simulink model "gm_sampleModel1420_3_sub"  (R2023a)
settings: Solver=VariableStepAuto  StartTime=0.0  StopTime=10.0  RelTol=1e-3
libraries: simulink x2, hdlsllib x2
settings Model: Creator=user1  LastModifiedBy=user1
settings OptimizationCC: BlockReduction=off  ConditionallyExecuteInputs=off
settings DebuggingCC: InheritedTsInSrcMsg=none

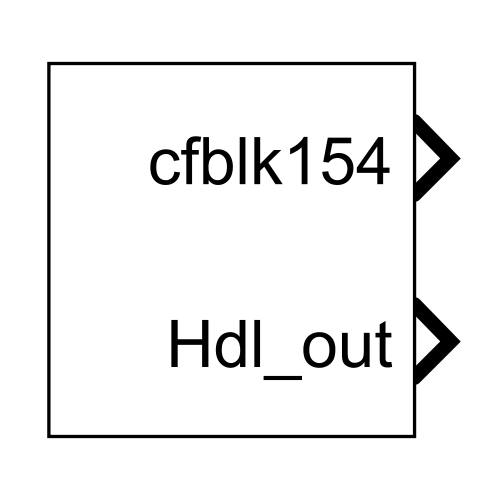
[thumbnail: Simulink's stored preview of the top-level diagram]
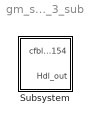
== system gm_sampleModel1420_3_sub ==
  Subsystem : Subsystem

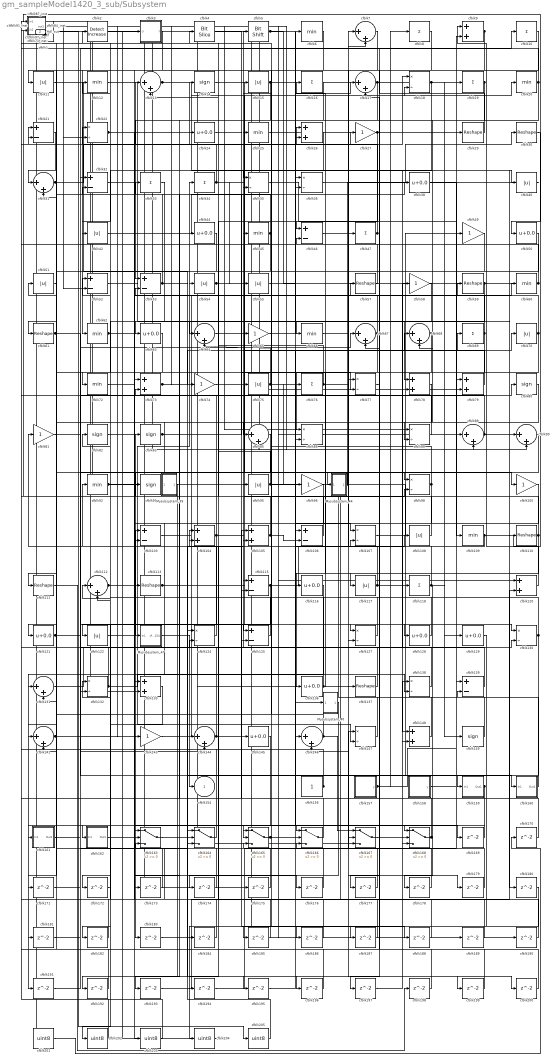
== system gm_sampleModel1420_3_sub/Subsystem ==
  Mysubsystem_39 : Subsystem
  Mysubsystem_40 : Subsystem
  Mysubsystem_44 : Subsystem
  Mysubsystem_47 : Subsystem
  cfblk1 : simulink/Logic and Bit Operations/Bit Clear  iBit=0
      settings: LibrarySourceBlock=|
      | hdlsllib/Logic and Bit
      | Operations/Bit Clear
  cfblk{8,10,16,19,33..34,47,69,76,118} (10 alike) : Sum  Inputs=+  OutDataTypeStr=uint8
  cfblk{27,49,58,65,74,81,96,100,143} (9 alike) : Gain  OutDataTypeStr=uint8
  cfblk102_inst : Subsystem
  cfblk{21,32,46,52..53,103,106,115,125,139} (10 alike) : Sum  Inputs=+-  OutDataTypeStr=uint8
  cfblk{9,26,73,78..79,104..105,120,133,148} (10 alike) : Sum  OutDataTypeStr=uint8
  cfblk{18,22,35..36,77,86,88,98,107,124,127,130,132,138,147} (15 alike) : Product  Inputs=*/  OutDataTypeStr=uint8  RndMeth=Zero  SaturateOnIntegerOverflow=on
  cfblk{11,15,40,42,51,54..55,70,75,95,108,117,122} (13 alike) : Abs  OutDataTypeStr=uint8  SaturateOnIntegerOverflow=off
  cfblk{6,12,20,25,45,60,62,66,72,92,109} (11 alike) : MinMax  OutDataTypeStr=uint8
  cfblk{29..30,57,59,61,110..111,113,137} (9 alike) : Reshape
  cfblk{7,13,17,31,64,67..68,85,89..90,112,131,141,144,146} (15 alike) : Sum  Inputs=|++  OutDataTypeStr=uint8
  cfblk114_inst : Subsystem
  cfblk{24,38,44,50,63,116,121,128..129,136,145} (11 alike) : Bias  Bias=0.0  SaturateOnIntegerOverflow=off
  cfblk119_inst : Subsystem
  cfblk135_inst : Subsystem
  cfblk{14,80,82..83,93,149} (6 alike) : Signum
  cfblk156 : Constant  OutDataTypeStr=uint8  SampleTime=-1
  cfblk157 : Subsystem  mask(Counter Limited){uplimit=double(7), tsamp=double(-1)}
      mask prompts: uplimit "Simulink:masks:UpperLimit_MP"; tsamp "Simulink:masks:SampleTime_MP"
      mask help: Simulink:masks:CounterLimited_MD
      mask init:
      | nbits = double(8);
      | tsamp = double(-1);
      | uplimit = double(7);
  cfblk158 : Subsystem  mask(Counter Free-Running){NumBits=double(16), tsamp=double(-1)}
      mask prompts: NumBits "Simulink:masks:NumberOfBits_MP"; tsamp "Simulink:masks:SampleTime_MP"
      mask help: Simulink:masks:CounterFreeRunning_MD
  cfblk159 : Subsystem
  cfblk160 : Subsystem
  cfblk161 : Subsystem
  cfblk162 : Subsystem
  cfblk{163..168} (6 alike) : Switch  OutDataTypeStr=uint8  SaturateOnIntegerOverflow=off  InputSameDT=off
  cfblk{169..200} (32 alike) : Delay  SampleTime=1
  cfblk2 : simulink/Logic and Bit Operations/Detect Increase  vinit=0.0  OutDataTypeStr=uint8
      settings: LibrarySourceBlock=|
      | hdlsllib/Logic and Bit
      | Operations/Detect
      | Increase
  cfblk{201..205} (5 alike) : DataTypeConversion  OutDataTypeStr=uint8  SaturateOnIntegerOverflow=off  RndMeth=Floor
  cfblk23_inst : Subsystem
  cfblk3 : Subsystem  mask(Detect Fall Negative){vinit=double(0), InputProcessing=Elements as channels (sample based), OutDataTypeStr=uint8}
      mask prompts: vinit "Simulink:masks:InitialCondition_MP"; InputProcessing "Simulink:masks:InputProcessing_MP"; OutDataTypeStr "Simulink:masks:OutputDataType_MP"
      mask help: Simulink:masks:DetectFallNegative_MD
      mask init:
      | InputProcessing = 'Elements as channels (sample based)';
      | OutDataTypeStr = 'uint8';
      | vinit = double(0);
      mask TypeOptions InputProcessing: Simulink:masks:ColumnsAsChannelsFrameBased | Simulink:masks:ElementsAsChannelsSampleBased
      mask TypeOptions OutDataTypeStr: Simulink:masks:uint8 | Simulink:masks:boolean
      mask Display: fprintf('U < 0\n&  NOT\nU/z < 0')
  cfblk4 : hdlsllib/Logic and Bit Operations/Bit Slice  lidx=7  ridx=0
  cfblk41_inst : Subsystem
  cfblk48_inst : Subsystem
  cfblk5 : hdlsllib/Logic and Bit Operations/Bit Shift  mode=Shift Left Logical  N=0
  cfblk56_inst : Subsystem
  cfblk71_inst : Subsystem
  cfblk84_inst : Subsystem
  cfblk87_inst : Subsystem
  cfblk91_inst : Subsystem
  cfblk97_inst : Subsystem
  cfblk154 : Outport  OutDataTypeStr=uint8  SampleTime=1  VectorParamsAs1DForOutWhenUnconnected=off
  Hdl_out : Outport  Port=2  OutDataTypeStr=uint8  SampleTime=1
  wires:
  Mysubsystem_39/1(Out1) -> cfblk192/1
  Mysubsystem_40/1(Out1) -> cfblk174/1
  Mysubsystem_44/1(Out1) -> cfblk183/1, cfblk159/1(In1)
  Mysubsystem_47/1(cfblk154) -> cfblk154/1
  cfblk1/1 -> cfblk205/1
  cfblk10/1 -> cfblk62/1
  cfblk100/1 -> cfblk143/1
  cfblk102_inst/1(out1) -> cfblk145/1, cfblk120/1
  cfblk103/1 -> cfblk57/1
  cfblk104/1 -> cfblk73/2, cfblk122/1, cfblk20/1
  cfblk105/1 -> cfblk5/1, cfblk106/2
  cfblk106/1 -> cfblk87_inst/2(in2)
  cfblk107/1 -> cfblk49/1
  cfblk108/1 -> cfblk52/1
  cfblk109/1 -> cfblk97_inst/1(in1), cfblk107/2
  cfblk11/1 -> cfblk164/2
  cfblk110/1 -> cfblk83/1, cfblk136/1
  cfblk111/1 -> cfblk198/1
  cfblk112/1 -> cfblk147/2, cfblk12/1, cfblk34/1
  cfblk113/1 -> cfblk128/1, cfblk98/2
  cfblk114_inst/1(out1) -> cfblk52/2
  cfblk115/1 -> cfblk7/2, cfblk162/1(In1)
  cfblk116/1 -> cfblk191/1
  cfblk117/1 -> cfblk58/1, cfblk2/1, cfblk92/1
  cfblk118/1 -> cfblk32/2, cfblk149/1, cfblk178/1
  cfblk119_inst/1(out1) -> cfblk201/1
  cfblk12/1 -> cfblk64/1
  cfblk120/1 -> cfblk9/1
  cfblk121/1 -> cfblk67/1, cfblk74/1
  cfblk122/1 -> cfblk103/1
  cfblk124/1 -> cfblk81/1
  cfblk125/1 -> cfblk71_inst/1(in1)
  cfblk127/1 -> cfblk87_inst/1(in1)
  cfblk128/1 -> cfblk106/1
  cfblk129/1 -> cfblk186/1
  cfblk13/1 -> cfblk180/1, cfblk18/2
  cfblk130/1 -> cfblk67/2, cfblk26/1, cfblk164/3
  cfblk131/1 -> cfblk78/2
  cfblk132/1 -> cfblk51/1, cfblk138/2
  cfblk133/1 -> cfblk172/1
  cfblk135_inst/1(out1) -> cfblk137/1
  cfblk136/1 -> cfblk95/1, cfblk200/1, cfblk16/1
  cfblk137/1 -> cfblk46/2
  cfblk138/1 -> cfblk82/1
  cfblk139/1 -> cfblk115/1
  cfblk14/1 -> cfblk148/1
  cfblk141/1 -> cfblk163/2, cfblk113/1
  cfblk143/1 -> cfblk47/1
  cfblk144/1 -> cfblk41_inst/2(in2), cfblk166/1
  cfblk145/1 -> cfblk202/1
  cfblk146/1 -> cfblk21/1, cfblk167/1, cfblk25/1
  cfblk147/1 -> cfblk102_inst/1(in1)
  cfblk148/1 -> cfblk104/1
  cfblk149/1 -> cfblk54/1
  cfblk15/1 -> cfblk40/1, cfblk193/1
  cfblk156/1 -> cfblk48_inst/2(in2), cfblk131/2
  cfblk157/1(y) -> cfblk9/2, cfblk8/1
  cfblk158/1(y) -> cfblk139/1
  cfblk159/1(Out1) -> cfblk182/1, cfblk181/1
  cfblk16/1 -> cfblk53/1
  cfblk160/1(Out1) -> cfblk139/2
  cfblk161/1(Out1) -> cfblk10/1
  cfblk162/1(Out1) -> cfblk27/1
  cfblk163/1 -> cfblk105/2
  cfblk164/1 -> cfblk84_inst/2(in2)
  cfblk165/1 -> cfblk70/1, cfblk108/1
  cfblk166/1 -> cfblk33/1
  cfblk167/1 -> cfblk138/1
  cfblk168/1 -> cfblk114_inst/2(in2), cfblk112/1
  cfblk169/1 -> cfblk165/2
  cfblk17/1 -> cfblk146/2, cfblk173/1
  cfblk170/1 -> cfblk105/1
  cfblk171/1 -> cfblk130/2
  cfblk172/1 -> cfblk132/1
  cfblk173/1 -> cfblk163/1
  cfblk174/1 -> cfblk112/2
  cfblk175/1 -> cfblk141/2
  cfblk176/1 -> cfblk124/2
  cfblk177/1 -> cfblk166/3
  cfblk178/1 -> cfblk147/1
  cfblk179/1 -> cfblk165/3
  cfblk18/1 -> cfblk42/1, cfblk129/1
  cfblk180/1 -> cfblk204/1
  cfblk181/1 -> cfblk144/2
  cfblk182/1 -> cfblk102_inst/2(in2)
  cfblk183/1 -> cfblk148/2
  cfblk184/1 -> cfblk163/3
  cfblk185/1 -> cfblk22/1
  cfblk186/1 -> cfblk84_inst/1(in1)
  cfblk187/1 -> cfblk26/2
  cfblk188/1 -> cfblk104/2
  cfblk189/1 -> cfblk73/1
  cfblk19/1 -> cfblk68/2, cfblk125/1
  cfblk190/1 -> cfblk21/2
  cfblk191/1 -> cfblk164/1
  cfblk192/1 -> cfblk23_inst/2(in2)
  cfblk193/1 -> cfblk120/2
  cfblk194/1 -> cfblk79/1
  cfblk195/1 -> cfblk146/1
  cfblk196/1 -> cfblk166/2
  cfblk197/1 -> cfblk168/3
  cfblk198/1 -> cfblk168/2
  cfblk199/1 -> cfblk17/2
  cfblk2/1 -> cfblk3/1(U)
  cfblk20/1 -> cfblk114_inst/1(in1), cfblk88/2
  cfblk200/1 -> cfblk31/2
  cfblk201/1 -> cfblk170/1
  cfblk202/1 -> cfblk119_inst/1(in1)
  cfblk203/1 -> cfblk119_inst/2(in2)
  cfblk204/1 -> cfblk1/1
  cfblk205/1 -> cfblk124/1
  cfblk21/1 -> cfblk31/1
  cfblk22/1 -> cfblk86/2, cfblk118/1
  cfblk23_inst/1(out1) -> cfblk167/3, cfblk144/1
  cfblk24/1 -> cfblk77/2
  cfblk25/1 -> Mysubsystem_40/1(In1)
  cfblk26/1 -> cfblk165/1
  cfblk27/1 -> cfblk46/1, cfblk184/1
  cfblk29/1 -> cfblk48_inst/1(in1)
  cfblk3/1(Y) -> cfblk203/1
  cfblk30/1 -> cfblk50/1
  cfblk31/1 -> cfblk7/1, cfblk14/1
  cfblk32/1 -> cfblk176/1
  cfblk33/1 -> cfblk63/1
  cfblk34/1 -> cfblk71_inst/2(in2), cfblk55/1, cfblk18/1
  cfblk35/1 -> cfblk89/1
  cfblk36/1 -> cfblk30/1
  cfblk38/1 -> cfblk109/1
  cfblk4/1 -> cfblk127/1
  cfblk40/1 -> Mysubsystem_39/1(In1)
  cfblk41_inst/1(out1) -> cfblk133/2
  cfblk42/1 -> cfblk6/1
  cfblk44/1 -> cfblk111/1
  cfblk45/1 -> cfblk97_inst/2(in2), cfblk103/2
  cfblk46/1 -> cfblk77/1
  cfblk47/1 -> cfblk91_inst/2(in2), cfblk13/1
  cfblk48_inst/1(out1) -> cfblk88/1, cfblk190/1
  cfblk49/1 -> cfblk187/1
  cfblk5/1 -> cfblk168/1, cfblk107/1
  cfblk50/1 -> cfblk85/1
  cfblk51/1 -> cfblk131/1
  cfblk52/1 -> cfblk110/1
  cfblk53/1 -> cfblk56_inst/1(in1), cfblk199/1
  cfblk54/1 -> cfblk38/1, cfblk188/1
  cfblk55/1 -> cfblk36/2
  cfblk56_inst/1(out1) -> cfblk90/1
  cfblk57/1 -> cfblk91_inst/1(in1)
  cfblk58/1 -> cfblk78/1
  cfblk59/1 -> cfblk197/1, cfblk72/1
  cfblk6/1 -> cfblk61/1
  cfblk60/1 -> cfblk41_inst/1(in1), Hdl_out/1
  cfblk61/1 -> cfblk160/1(In1), Mysubsystem_47/1(In1), Mysubsystem_44/1(In1)
  cfblk62/1 -> cfblk130/1, cfblk60/1
  cfblk63/1 -> cfblk161/1(In1)
  cfblk64/1 -> cfblk66/1
  cfblk65/1 -> cfblk17/1
  cfblk66/1 -> cfblk169/1
  cfblk67/1 -> cfblk15/1, cfblk115/2
  cfblk68/1 -> cfblk116/1, cfblk86/1
  cfblk69/1 -> cfblk4/1, cfblk35/2, cfblk194/1
  cfblk7/1 -> cfblk185/1
  cfblk70/1 -> cfblk53/2, cfblk141/1
  cfblk71_inst/1(out1) -> cfblk85/2, cfblk29/1, cfblk22/2
  cfblk72/1 -> cfblk196/1
  cfblk73/1 -> cfblk195/1, cfblk69/1
  cfblk74/1 -> cfblk68/1
  cfblk75/1 -> cfblk64/2, cfblk96/1
  cfblk76/1 -> cfblk13/2, cfblk179/1
  cfblk77/1 -> cfblk177/1
  cfblk78/1 -> cfblk171/1
  cfblk79/1 -> cfblk65/1
  cfblk8/1 -> cfblk117/1
  cfblk80/1 -> cfblk93/1
  cfblk81/1 -> cfblk80/1
  cfblk82/1 -> cfblk75/1
  cfblk83/1 -> cfblk59/1, cfblk36/1
  cfblk84_inst/1(out1) -> cfblk90/2, cfblk79/2
  cfblk85/1 -> cfblk121/1
  cfblk86/1 -> cfblk100/1
  cfblk87_inst/1(out1) -> cfblk89/2, cfblk175/1, cfblk19/1
  cfblk88/1 -> cfblk45/1
  cfblk89/1 -> cfblk56_inst/2(in2), cfblk32/1, cfblk135_inst/2(in2)
  cfblk9/1 -> cfblk11/1, cfblk35/1, cfblk127/2
  cfblk90/1 -> cfblk132/2
  cfblk91_inst/1(out1) -> cfblk189/1
  cfblk92/1 -> cfblk24/1, cfblk167/2
  cfblk93/1 -> cfblk23_inst/1(in1)
  cfblk95/1 -> cfblk44/1, cfblk98/1
  cfblk96/1 -> cfblk133/1
  cfblk97_inst/1(out1) -> cfblk76/1
  cfblk98/1 -> cfblk135_inst/1(in1), cfblk125/2

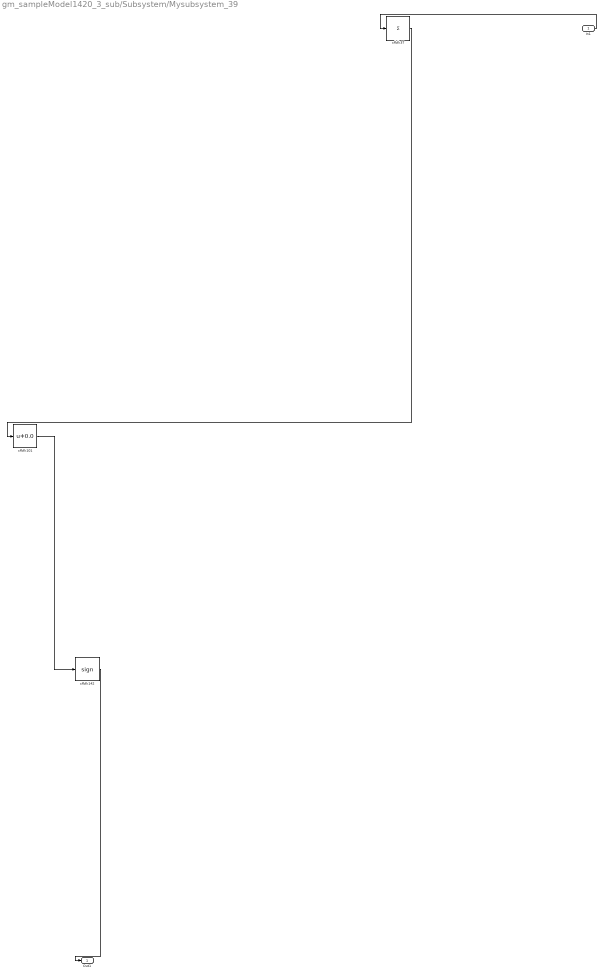
== system gm_sampleModel1420_3_sub/Subsystem/Mysubsystem_39 ==
  In1 : Inport  OutDataTypeStr=uint8  PortDimensions=1  SampleTime=1
  cfblk101 : Bias  Bias=0.0  SaturateOnIntegerOverflow=off
  cfblk142 : Signum
  cfblk37 : Sum  Inputs=+
  Out1 : Outport  SampleTime=1
  wires:
  In1/1 -> cfblk37/1
  cfblk101/1 -> cfblk142/1
  cfblk142/1 -> Out1/1
  cfblk37/1 -> cfblk101/1

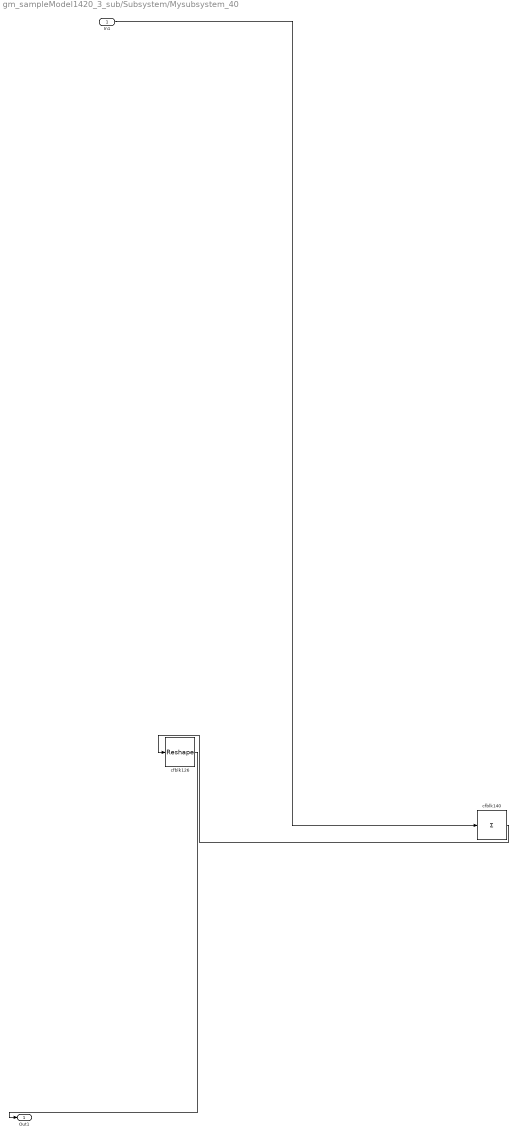
== system gm_sampleModel1420_3_sub/Subsystem/Mysubsystem_40 ==
  In1 : Inport  OutDataTypeStr=uint8  PortDimensions=1  SampleTime=1
  cfblk126 : Reshape
  cfblk140 : Sum  Inputs=+
  Out1 : Outport  SampleTime=1
  wires:
  In1/1 -> cfblk140/1
  cfblk126/1 -> Out1/1
  cfblk140/1 -> cfblk126/1

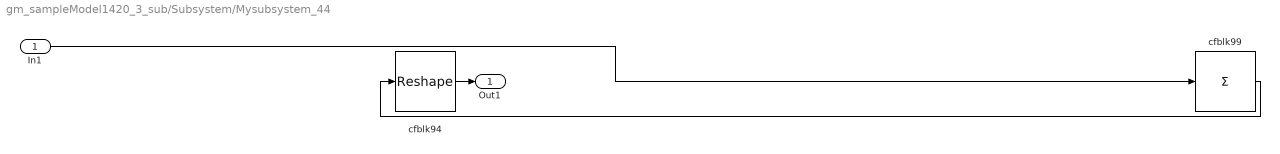
== system gm_sampleModel1420_3_sub/Subsystem/Mysubsystem_44 ==
  In1 : Inport  OutDataTypeStr=uint8  PortDimensions=1  SampleTime=1
  cfblk94 : Reshape
  cfblk99 : Sum  Inputs=+
  Out1 : Outport  SampleTime=1
  wires:
  In1/1 -> cfblk99/1
  cfblk94/1 -> Out1/1
  cfblk99/1 -> cfblk94/1

== system gm_sampleModel1420_3_sub/Subsystem/Mysubsystem_47 ==
  In1 : Inport  OutDataTypeStr=uint8  PortDimensions=1  SampleTime=1
  cfblk123 : Abs  SaturateOnIntegerOverflow=off
  cfblk154 : Outport  SampleTime=1  VectorParamsAs1DForOutWhenUnconnected=off
  wires:
  In1/1 -> cfblk123/1
  cfblk123/1 -> cfblk154/1

== system gm_sampleModel1420_3_sub/Subsystem/cfblk102_inst ==
  in1 : Inport  OutDataTypeStr=uint8  SampleTime=1
  in2 : Inport  Port=2  OutDataTypeStr=uint8  SampleTime=1
  mul_cfblk102_dotp_mulcomp : Product  Inputs=**  OutDataTypeStr=uint8  SampleTime=1
  out1 : Outport  OutDataTypeStr=uint8  SampleTime=1
  wires:
  in1/1 -> mul_cfblk102_dotp_mulcomp/1
  in2/1 -> mul_cfblk102_dotp_mulcomp/2
  mul_cfblk102_dotp_mulcomp/1 -> out1/1

== system gm_sampleModel1420_3_sub/Subsystem/cfblk114_inst ==
  in1 : Inport  OutDataTypeStr=uint8  SampleTime=1
  in2 : Inport  Port=2  OutDataTypeStr=uint8  SampleTime=1
  mul_cfblk114_dotp_mulcomp : Product  Inputs=**  OutDataTypeStr=uint8  SampleTime=1
  out1 : Outport  OutDataTypeStr=uint8  SampleTime=1
  wires:
  in1/1 -> mul_cfblk114_dotp_mulcomp/1
  in2/1 -> mul_cfblk114_dotp_mulcomp/2
  mul_cfblk114_dotp_mulcomp/1 -> out1/1

== system gm_sampleModel1420_3_sub/Subsystem/cfblk119_inst ==
  in1 : Inport  OutDataTypeStr=uint8  SampleTime=1
  in2 : Inport  Port=2  OutDataTypeStr=uint8  SampleTime=1
  mul_cfblk119_dotp_mulcomp : Product  Inputs=**  OutDataTypeStr=uint8  SampleTime=1
  out1 : Outport  OutDataTypeStr=uint8  SampleTime=1
  wires:
  in1/1 -> mul_cfblk119_dotp_mulcomp/1
  in2/1 -> mul_cfblk119_dotp_mulcomp/2
  mul_cfblk119_dotp_mulcomp/1 -> out1/1

== system gm_sampleModel1420_3_sub/Subsystem/cfblk135_inst ==
  in1 : Inport  OutDataTypeStr=uint8  SampleTime=1
  in2 : Inport  Port=2  OutDataTypeStr=uint8  SampleTime=1
  mul_cfblk135_dotp_mulcomp : Product  Inputs=**  OutDataTypeStr=uint8  SampleTime=1
  out1 : Outport  OutDataTypeStr=uint8  SampleTime=1
  wires:
  in1/1 -> mul_cfblk135_dotp_mulcomp/1
  in2/1 -> mul_cfblk135_dotp_mulcomp/2
  mul_cfblk135_dotp_mulcomp/1 -> out1/1

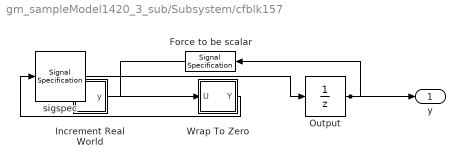
== system gm_sampleModel1420_3_sub/Subsystem/cfblk157 ==
  Force to be scalar : SignalSpecification  DisableCoverage=on  Dimensions=1
  Increment Real World : Subsystem  mask(Real World Value Increment){}
      mask help: Simulink:masks:RealWorldValueIncrement_MD
      mask Display: disp('V++')
  Output : UnitDelay  InitialCondition=0.0  SampleTime=tsamp  HasFrameUpgradeWarning=on
  Wrap To Zero : Subsystem  mask(Wrap To Zero){Threshold=double(7)}
      mask prompts: Threshold "Simulink:masks:Threshold_MP"
      mask help: Simulink:masks:WrapToZero_MD
  sigspec : SignalSpecification  OutDataTypeStr=uint8  Dimensions=1
  y : Outport  SampleTime=1
  wires:
  Force to be scalar/1 -> Increment Real World/1(u)
  Increment Real World/1(y) -> Wrap To Zero/1(U)
  Output/1 -> Force to be scalar/1, y/1
  Wrap To Zero/1(Y) -> sigspec/1
  sigspec/1 -> Output/1

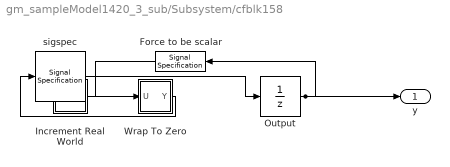
== system gm_sampleModel1420_3_sub/Subsystem/cfblk158 ==
  Force to be scalar : SignalSpecification  DisableCoverage=on  Dimensions=1
  Increment Real World : Subsystem  mask(Real World Value Increment){}
      mask help: Simulink:masks:RealWorldValueIncrement_MD
      mask Display: disp('V++')
  Output : UnitDelay  InitialCondition=0.0  SampleTime=tsamp  HasFrameUpgradeWarning=on
  Wrap To Zero : Subsystem  mask(Wrap To Zero){Threshold=double(65535)}
      mask prompts: Threshold "Simulink:masks:Threshold_MP"
      mask help: Simulink:masks:WrapToZero_MD
  sigspec : SignalSpecification  OutDataTypeStr=uint16  Dimensions=1
  y : Outport  SampleTime=1
  wires:
  Force to be scalar/1 -> Increment Real World/1(u)
  Increment Real World/1(y) -> Wrap To Zero/1(U)
  Output/1 -> Force to be scalar/1, y/1
  Wrap To Zero/1(Y) -> sigspec/1
  sigspec/1 -> Output/1

== system gm_sampleModel1420_3_sub/Subsystem/cfblk159 ==
  In1 : Inport  OutDataTypeStr=uint8  PortDimensions=1  SampleTime=1
  Out1 : Outport  SampleTime=1
  wires:
  In1/1 -> Out1/1

== system gm_sampleModel1420_3_sub/Subsystem/cfblk160 ==
  In1 : Inport  OutDataTypeStr=uint8  PortDimensions=1  SampleTime=1
  Out1 : Outport  SampleTime=1
  wires:
  In1/1 -> Out1/1

== system gm_sampleModel1420_3_sub/Subsystem/cfblk161 ==
  In1 : Inport  OutDataTypeStr=uint8  PortDimensions=1  SampleTime=1
  Out1 : Outport  SampleTime=1
  wires:
  In1/1 -> Out1/1

== system gm_sampleModel1420_3_sub/Subsystem/cfblk162 ==
  In1 : Inport  OutDataTypeStr=uint8  PortDimensions=1  SampleTime=1
  Out1 : Outport  SampleTime=1
  wires:
  In1/1 -> Out1/1

== system gm_sampleModel1420_3_sub/Subsystem/cfblk23_inst ==
  in1 : Inport  OutDataTypeStr=uint8  SampleTime=1
  in2 : Inport  Port=2  OutDataTypeStr=uint8  SampleTime=1
  mul_cfblk23_dotp_mulcomp : Product  Inputs=**  OutDataTypeStr=uint8  SampleTime=1
  out1 : Outport  OutDataTypeStr=uint8  SampleTime=1
  wires:
  in1/1 -> mul_cfblk23_dotp_mulcomp/1
  in2/1 -> mul_cfblk23_dotp_mulcomp/2
  mul_cfblk23_dotp_mulcomp/1 -> out1/1

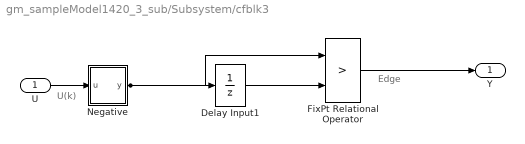
== system gm_sampleModel1420_3_sub/Subsystem/cfblk3 ==
  note: U(k)
  note: Edge
  U : Inport  OutDataTypeStr=uint8  SampleTime=1
  Delay Input1 : UnitDelay  Description=Store in Global RAM  DisableCoverage=on  InitialCondition=vinit  SampleTime=-1  HasFrameUpgradeWarning=on
  FixPt Relational Operator : RelationalOperator  Operator=>  OutDataTypeStr=fixdt(0, 8)  ZeroCross=off  InputSameDT=off
  Negative : Subsystem  mask(Compare To Zero){relop=<, OutDataTypeStr=boolean, ZeroCross=off}
      mask prompts: relop "Simulink:masks:Operator_MP"; OutDataTypeStr "Simulink:masks:OutputDataType_MP"; ZeroCross "Simulink:masks:EnableZerocrossingDetection_MP"
      mask help: Simulink:masks:CompareToZero_MD
      mask init:
      | OutDataTypeStr = 'boolean';
      | ZeroCross = 'off';
      | blkName = 'sampleModel1420_3_sub/Subsystem/cfblk3/Negative';
      | relop = '<';
      | setValue = 'boolean';
      mask TypeOptions relop: == | ~= | < | <= | >= | >
      mask TypeOptions OutDataTypeStr: Simulink:masks:uint8 | Simulink:masks:boolean
      mask Callback ZeroCross: sl('zeroCrossEnable', gcbh);
      mask Display: disp([relop,' 0'])
  Y : Outport  SampleTime=1
  wires:
  U/1 -> Negative/1(u)
  Delay Input1/1 -> FixPt Relational Operator/2
  FixPt Relational Operator/1 -> Y/1
  Negative/1(y) -> FixPt Relational Operator/1, Delay Input1/1

== system gm_sampleModel1420_3_sub/Subsystem/cfblk41_inst ==
  in1 : Inport  OutDataTypeStr=uint8  SampleTime=1
  in2 : Inport  Port=2  OutDataTypeStr=uint8  SampleTime=1
  mul_cfblk41_dotp_mulcomp : Product  Inputs=**  OutDataTypeStr=uint8  SampleTime=1
  out1 : Outport  OutDataTypeStr=uint8  SampleTime=1
  wires:
  in1/1 -> mul_cfblk41_dotp_mulcomp/1
  in2/1 -> mul_cfblk41_dotp_mulcomp/2
  mul_cfblk41_dotp_mulcomp/1 -> out1/1

== system gm_sampleModel1420_3_sub/Subsystem/cfblk48_inst ==
  in1 : Inport  OutDataTypeStr=uint8  SampleTime=1
  in2 : Inport  Port=2  OutDataTypeStr=uint8  SampleTime=1
  mul_cfblk48_dotp_mulcomp : Product  Inputs=**  OutDataTypeStr=uint8  SampleTime=1
  out1 : Outport  OutDataTypeStr=uint8  SampleTime=1
  wires:
  in1/1 -> mul_cfblk48_dotp_mulcomp/1
  in2/1 -> mul_cfblk48_dotp_mulcomp/2
  mul_cfblk48_dotp_mulcomp/1 -> out1/1

== system gm_sampleModel1420_3_sub/Subsystem/cfblk56_inst ==
  in1 : Inport  OutDataTypeStr=uint8  SampleTime=1
  in2 : Inport  Port=2  OutDataTypeStr=uint8  SampleTime=1
  mul_cfblk56_dotp_mulcomp : Product  Inputs=**  OutDataTypeStr=uint8  SampleTime=1
  out1 : Outport  OutDataTypeStr=uint8  SampleTime=1
  wires:
  in1/1 -> mul_cfblk56_dotp_mulcomp/1
  in2/1 -> mul_cfblk56_dotp_mulcomp/2
  mul_cfblk56_dotp_mulcomp/1 -> out1/1

== system gm_sampleModel1420_3_sub/Subsystem/cfblk71_inst ==
  in1 : Inport  OutDataTypeStr=uint8  SampleTime=1
  in2 : Inport  Port=2  OutDataTypeStr=uint8  SampleTime=1
  mul_cfblk71_dotp_mulcomp : Product  Inputs=**  OutDataTypeStr=uint8  SampleTime=1
  out1 : Outport  OutDataTypeStr=uint8  SampleTime=1
  wires:
  in1/1 -> mul_cfblk71_dotp_mulcomp/1
  in2/1 -> mul_cfblk71_dotp_mulcomp/2
  mul_cfblk71_dotp_mulcomp/1 -> out1/1

== system gm_sampleModel1420_3_sub/Subsystem/cfblk84_inst ==
  in1 : Inport  OutDataTypeStr=uint8  SampleTime=1
  in2 : Inport  Port=2  OutDataTypeStr=uint8  SampleTime=1
  mul_cfblk84_dotp_mulcomp : Product  Inputs=**  OutDataTypeStr=uint8  SampleTime=1
  out1 : Outport  OutDataTypeStr=uint8  SampleTime=1
  wires:
  in1/1 -> mul_cfblk84_dotp_mulcomp/1
  in2/1 -> mul_cfblk84_dotp_mulcomp/2
  mul_cfblk84_dotp_mulcomp/1 -> out1/1

== system gm_sampleModel1420_3_sub/Subsystem/cfblk87_inst ==
  in1 : Inport  OutDataTypeStr=uint8  SampleTime=1
  in2 : Inport  Port=2  OutDataTypeStr=uint8  SampleTime=1
  mul_cfblk87_dotp_mulcomp : Product  Inputs=**  OutDataTypeStr=uint8  SampleTime=1
  out1 : Outport  OutDataTypeStr=uint8  SampleTime=1
  wires:
  in1/1 -> mul_cfblk87_dotp_mulcomp/1
  in2/1 -> mul_cfblk87_dotp_mulcomp/2
  mul_cfblk87_dotp_mulcomp/1 -> out1/1

== system gm_sampleModel1420_3_sub/Subsystem/cfblk91_inst ==
  in1 : Inport  OutDataTypeStr=uint8  SampleTime=1
  in2 : Inport  Port=2  OutDataTypeStr=uint8  SampleTime=1
  mul_cfblk91_dotp_mulcomp : Product  Inputs=**  OutDataTypeStr=uint8  SampleTime=1
  out1 : Outport  OutDataTypeStr=uint8  SampleTime=1
  wires:
  in1/1 -> mul_cfblk91_dotp_mulcomp/1
  in2/1 -> mul_cfblk91_dotp_mulcomp/2
  mul_cfblk91_dotp_mulcomp/1 -> out1/1

== system gm_sampleModel1420_3_sub/Subsystem/cfblk97_inst ==
  in1 : Inport  OutDataTypeStr=uint8  SampleTime=1
  in2 : Inport  Port=2  OutDataTypeStr=uint8  SampleTime=1
  mul_cfblk97_dotp_mulcomp : Product  Inputs=**  OutDataTypeStr=uint8  SampleTime=1
  out1 : Outport  OutDataTypeStr=uint8  SampleTime=1
  wires:
  in1/1 -> mul_cfblk97_dotp_mulcomp/1
  in2/1 -> mul_cfblk97_dotp_mulcomp/2
  mul_cfblk97_dotp_mulcomp/1 -> out1/1

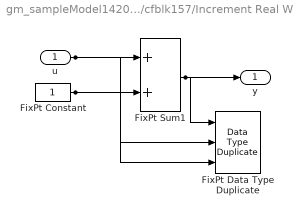
== system gm_sampleModel1420_3_sub/Subsystem/cfblk157/Increment Real World ==
  u : Inport  OutDataTypeStr=uint8  SampleTime=1
  FixPt Constant : Constant  DisableCoverage=on  OutDataTypeStr=Inherit: Inherit via back propagation  SampleTime=-1
  FixPt Data Type Duplicate : DataTypeDuplicate  DisableCoverage=on  NumInputPorts=3
  FixPt Sum1 : Sum  InputSameDT=on  OutDataTypeStr=Inherit: Inherit via back propagation  LockScale=on
  y : Outport  SampleTime=1
  wires:
  u/1 -> FixPt Sum1/1, FixPt Data Type Duplicate/2
  FixPt Constant/1 -> FixPt Sum1/2, FixPt Data Type Duplicate/3
  FixPt Sum1/1 -> FixPt Data Type Duplicate/1, y/1

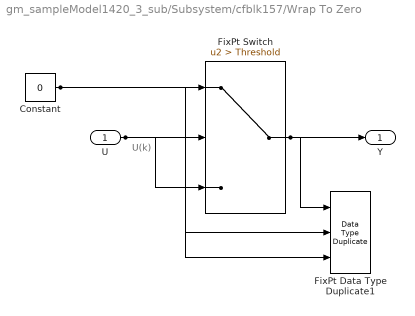
== system gm_sampleModel1420_3_sub/Subsystem/cfblk157/Wrap To Zero ==
  note: U(k)
  U : Inport  OutDataTypeStr=uint8  SampleTime=1
  Constant : Constant  DisableCoverage=on  Value=0  OutDataTypeStr=Inherit: Inherit via back propagation  SampleTime=-1
  FixPt Data Type Duplicate1 : DataTypeDuplicate  DisableCoverage=on  NumInputPorts=3
  FixPt Switch : Switch  Criteria=u2 > Threshold  Threshold=Threshold  OutDataTypeStr=Inherit: Inherit via back propagation  ZeroCross=off  SaturateOnIntegerOverflow=off  InputSameDT=off
  Y : Outport  SampleTime=1
  wires:
  U/1 -> FixPt Switch/3, FixPt Switch/2, FixPt Data Type Duplicate1/2
  Constant/1 -> FixPt Switch/1, FixPt Data Type Duplicate1/3
  FixPt Switch/1 -> FixPt Data Type Duplicate1/1, Y/1

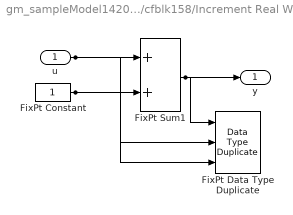
== system gm_sampleModel1420_3_sub/Subsystem/cfblk158/Increment Real World ==
  u : Inport  OutDataTypeStr=uint16  SampleTime=1
  FixPt Constant : Constant  DisableCoverage=on  OutDataTypeStr=Inherit: Inherit via back propagation  SampleTime=-1
  FixPt Data Type Duplicate : DataTypeDuplicate  DisableCoverage=on  NumInputPorts=3
  FixPt Sum1 : Sum  InputSameDT=on  OutDataTypeStr=Inherit: Inherit via back propagation  LockScale=on
  y : Outport  SampleTime=1
  wires:
  u/1 -> FixPt Sum1/1, FixPt Data Type Duplicate/2
  FixPt Constant/1 -> FixPt Sum1/2, FixPt Data Type Duplicate/3
  FixPt Sum1/1 -> FixPt Data Type Duplicate/1, y/1

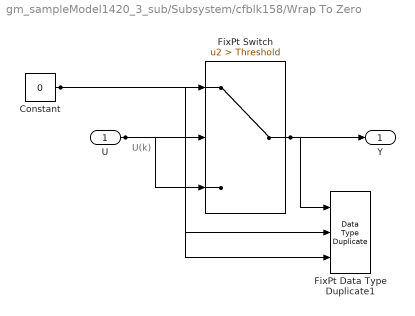
== system gm_sampleModel1420_3_sub/Subsystem/cfblk158/Wrap To Zero ==
  note: U(k)
  U : Inport  OutDataTypeStr=uint16  SampleTime=1
  Constant : Constant  DisableCoverage=on  Value=0  OutDataTypeStr=Inherit: Inherit via back propagation  SampleTime=-1
  FixPt Data Type Duplicate1 : DataTypeDuplicate  DisableCoverage=on  NumInputPorts=3
  FixPt Switch : Switch  Criteria=u2 > Threshold  Threshold=Threshold  OutDataTypeStr=Inherit: Inherit via back propagation  ZeroCross=off  SaturateOnIntegerOverflow=off  InputSameDT=off
  Y : Outport  SampleTime=1
  wires:
  U/1 -> FixPt Switch/3, FixPt Switch/2, FixPt Data Type Duplicate1/2
  Constant/1 -> FixPt Switch/1, FixPt Data Type Duplicate1/3
  FixPt Switch/1 -> FixPt Data Type Duplicate1/1, Y/1

== system gm_sampleModel1420_3_sub/Subsystem/cfblk3/Negative ==
  u : Inport  OutDataTypeStr=uint8  SampleTime=1
  Compare : RelationalOperator  Operator=<  OutDataTypeStr=boolean  ZeroCross=off
  Constant : Constant  DisableCoverage=on  Value=0  OutDataTypeStr=Inherit: Inherit via back propagation  SampleTime=-1  PreserveConstantTs=on
  y : Outport  SampleTime=1
  wires:
  u/1 -> Compare/1
  Compare/1 -> y/1
  Constant/1 -> Compare/2
